simulink model "linear_sim_with_control"  (R2024b)
settings: Solver=ode45  StartTime=0.0  StopTime=3  RelTol=1e-3
values from neighbouring files (symbols this model uses):
  C_rate = minreal(tf([0.0032072, 0.0353636, 0.01688], [0.00048, 1, 0]))    [linear_plants.m]
  G_rate = minreal(tf([-0.017463471379055, 11.6423142527021, -2587.18094504468, 191643.032966257],      [1, 35.9182674299634, 622.376679243638, 0]))    [linear_plants.m]
settings Model: Creator=tommy  LastModifiedBy=tommy

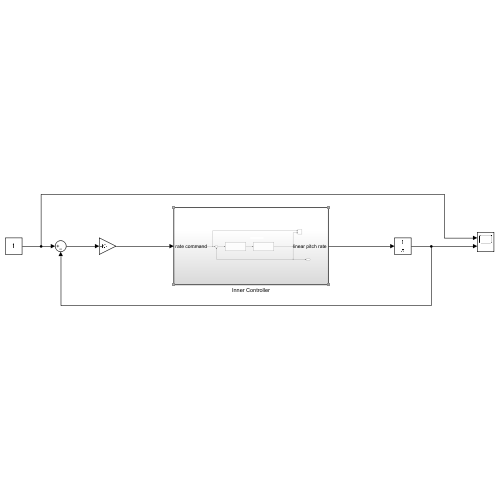
[thumbnail: Simulink's stored preview of the top-level diagram]
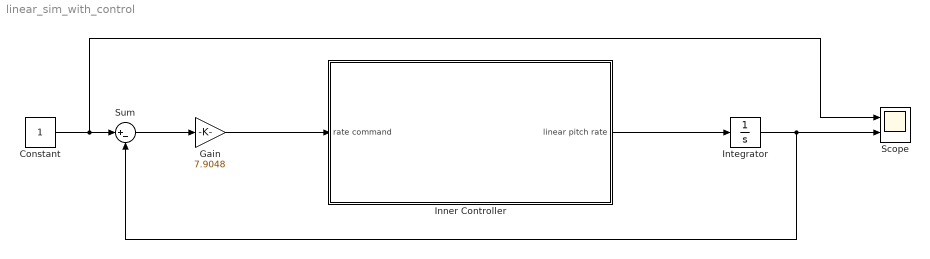
== system linear_sim_with_control ==
  Constant : Constant
  Gain : Gain  Gain=7.9048
  Inner Controller : Subsystem
  Integrator : Integrator
  Scope : Scope  NumInputPorts=2
  Sum : Sum  Inputs=|+-
  wires:
  Gain/1 -> Inner Controller/1(rate command)
  Integrator/1 -> Sum/2, Scope/2
  Inner Controller/1(linear pitch rate) -> Integrator/1
  Sum/1 -> Gain/1
  Constant/1 -> Scope/1, Sum/1

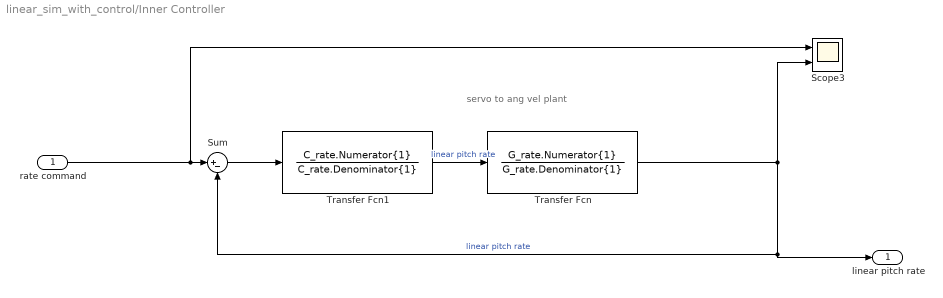
== system linear_sim_with_control/Inner Controller ==
  note: servo to ang vel plant
  rate command : Inport
  Scope3 : Scope  NumInputPorts=2
  Sum : Sum  Inputs=|+-
  Transfer Fcn : TransferFcn  Numerator=G_rate.Numerator{1}  Denominator=G_rate.Denominator{1}
  Transfer Fcn1 : TransferFcn  Numerator=C_rate.Numerator{1}  Denominator=C_rate.Denominator{1}
  linear pitch rate : Outport
  wires:
  Transfer Fcn/1 -> linear pitch rate/1, Sum/2, Scope3/2  "linear pitch rate"
  Sum/1 -> Transfer Fcn1/1
  Transfer Fcn1/1 -> Transfer Fcn/1  "linear pitch rate"
  rate command/1 -> Scope3/1, Sum/1
